simulink model "wlan_agc"  (Simulink 7.8)
settings: Solver=VariableStepDiscrete  SolverMode=SingleTasking  StartTime=0.0  StopTime=1e4  RelTol=1e-3
PostLoadFcn:
  | wlan_agc_init
InitFcn:
  | wlan_agc_init
StartFcn:
  | wlan_agc_init
values from neighbouring files (symbols this model uses):
  PHY_CONFIG_PKT_DET_CORR_THRESH = 90    [wlan_agc_init.m]
  PHY_CONFIG_PKT_DET_ENERGY_THRESH = 1    [wlan_agc_init.m]
  PHY_CONFIG_PKT_DET_MIN_DURR = 4    [wlan_agc_init.m]
undefined symbols (not defined in the file or in its folder): gcbh, xlBlockLoadCallback, xlGetNormalizedPeriod
libraries: xbsIndex_r4 x991, xbsEDKLib_r4 x1, simulink x1
(part 3 of 7)

== system wlan_agc/Gain Calc A ==
  I : Inport
  Q : Inport  Port=2
  IQ Valid : Inport  Port=3
  RSSI : Inport  Port=4
  BB gain : Subsystem
  Capture & Convert : Subsystem
  IQ Mag : Subsystem
  RF Gain : Subsystem
  RSSI Avg : Subsystem
  Register{1..4} (4 alike) : xbsIndex_r4/Register  init=0  rst=off  en=off  dbl_ovrd=off  block_type=register
  G_RF : Outport
  G_BB : Outport  Port=2
  wires:
  RF Gain/1(G_RF) -> Register1/1, Capture & Convert/1(G_RF)
  Register1/1 -> Register2/1
  RSSI/1 -> RSSI Avg/1(RSSI)
  RSSI Avg/1(avg) -> Capture & Convert/2(RSSI)
  Capture & Convert/1(Rx Pwr (dBm)) -> RF Gain/1(Rx Pwr), BB gain/2(P_IN_RSSI)
  Register3/1 -> Register4/1
  BB gain/1(G_BB) -> Register3/1
  RF Gain/2(G_RF_dB) -> BB gain/1(G_RF_dB)
  IQ Mag/1(IQ_dBv) -> BB gain/3(IQ_dBv)
  I/1 -> IQ Mag/1(I)
  Q/1 -> IQ Mag/2(Q)
  IQ Valid/1 -> IQ Mag/3(Valid)
  Register2/1 -> G_RF/1
  Register4/1 -> G_BB/1

== system wlan_agc/Gain Calc B ==
  I : Inport
  Q : Inport  Port=2
  IQ Valid : Inport  Port=3
  RSSI : Inport  Port=4
  BB gain : Subsystem
  Capture & Convert : Subsystem
  IQ Mag : Subsystem
  RF Gain : Subsystem
  RSSI Avg : Subsystem
  Register{1..4} (4 alike) : xbsIndex_r4/Register  init=0  rst=off  en=off  dbl_ovrd=off  block_type=register
  G_RF : Outport
  G_BB : Outport  Port=2
  wires:
  Register4/1 -> G_BB/1
  Register2/1 -> G_RF/1
  IQ Valid/1 -> IQ Mag/3(Valid)
  Q/1 -> IQ Mag/2(Q)
  I/1 -> IQ Mag/1(I)
  IQ Mag/1(IQ_dBv) -> BB gain/3(IQ_dBv)
  RF Gain/2(G_RF_dB) -> BB gain/1(G_RF_dB)
  BB gain/1(G_BB) -> Register3/1
  Register3/1 -> Register4/1
  Capture & Convert/1(Rx Pwr (dBm)) -> BB gain/2(P_IN_RSSI), RF Gain/1(Rx Pwr)
  RSSI Avg/1(avg) -> Capture & Convert/2(RSSI)
  RSSI/1 -> RSSI Avg/1(RSSI)
  Register1/1 -> Register2/1
  RF Gain/1(G_RF) -> Capture & Convert/1(G_RF), Register1/1

== system wlan_agc/Gain Calc C ==
  I : Inport
  Q : Inport  Port=2
  IQ Valid : Inport  Port=3
  RSSI : Inport  Port=4
  BB gain : Subsystem
  Capture & Convert : Subsystem
  IQ Mag : Subsystem
  RF Gain : Subsystem
  RSSI Avg : Subsystem
  Register{1..4} (4 alike) : xbsIndex_r4/Register  init=0  rst=off  en=off  dbl_ovrd=off  block_type=register
  G_RF : Outport
  G_BB : Outport  Port=2
  wires:
  RF Gain/1(G_RF) -> Register1/1, Capture & Convert/1(G_RF)
  Register1/1 -> Register2/1
  RSSI/1 -> RSSI Avg/1(RSSI)
  RSSI Avg/1(avg) -> Capture & Convert/2(RSSI)
  Capture & Convert/1(Rx Pwr (dBm)) -> RF Gain/1(Rx Pwr), BB gain/2(P_IN_RSSI)
  Register3/1 -> Register4/1
  BB gain/1(G_BB) -> Register3/1
  RF Gain/2(G_RF_dB) -> BB gain/1(G_RF_dB)
  IQ Mag/1(IQ_dBv) -> BB gain/3(IQ_dBv)
  I/1 -> IQ Mag/1(I)
  Q/1 -> IQ Mag/2(Q)
  IQ Valid/1 -> IQ Mag/3(Valid)
  Register2/1 -> G_RF/1
  Register4/1 -> G_BB/1

== system wlan_agc/Gain Calc D ==
  I : Inport
  Q : Inport  Port=2
  IQ Valid : Inport  Port=3
  RSSI : Inport  Port=4
  BB gain : Subsystem
  Capture & Convert : Subsystem
  IQ Mag : Subsystem
  RF Gain : Subsystem
  RSSI Avg : Subsystem
  Register{1..4} (4 alike) : xbsIndex_r4/Register  init=0  rst=off  en=off  dbl_ovrd=off  block_type=register
  G_RF : Outport
  G_BB : Outport  Port=2
  wires:
  Register4/1 -> G_BB/1
  Register2/1 -> G_RF/1
  IQ Valid/1 -> IQ Mag/3(Valid)
  Q/1 -> IQ Mag/2(Q)
  I/1 -> IQ Mag/1(I)
  IQ Mag/1(IQ_dBv) -> BB gain/3(IQ_dBv)
  RF Gain/2(G_RF_dB) -> BB gain/1(G_RF_dB)
  BB gain/1(G_BB) -> Register3/1
  Register3/1 -> Register4/1
  Capture & Convert/1(Rx Pwr (dBm)) -> BB gain/2(P_IN_RSSI), RF Gain/1(Rx Pwr)
  RSSI Avg/1(avg) -> Capture & Convert/2(RSSI)
  RSSI/1 -> RSSI Avg/1(RSSI)
  Register1/1 -> Register2/1
  RF Gain/1(G_RF) -> Capture & Convert/1(G_RF), Register1/1

== system wlan_agc/IQ Outputs ==
  IQ Valid : Inport
  A I : Inport  Port=2
  A Q : Inport  Port=3
  B I : Inport  Port=4
  B Q : Inport  Port=5
  C I : Inport  Port=6
  C Q : Inport  Port=7
  D I : Inport  Port=8
  D Q : Inport  Port=9
  IQ_Valid_Out : xbsIndex_r4/Gateway Out  inherit_from_input=off  hdl_port=on  timing_constraint=None  locs_specified=off  LOCs={}  UseAsDAC=off  DACChannel='1'  block_type=gatewayout
  RFA_RX_I_OUT : xbsIndex_r4/Gateway Out  inherit_from_input=off  hdl_port=on  timing_constraint=None  locs_specified=off  LOCs={}  UseAsDAC=off  DACChannel='1'  block_type=gatewayout
  RFA_RX_Q_OUT : xbsIndex_r4/Gateway Out  inherit_from_input=off  hdl_port=on  timing_constraint=None  locs_specified=off  LOCs={}  UseAsDAC=off  DACChannel='1'  block_type=gatewayout
  RFB_RX_I_OUT : xbsIndex_r4/Gateway Out  inherit_from_input=off  hdl_port=on  timing_constraint=None  locs_specified=off  LOCs={}  UseAsDAC=off  DACChannel='1'  block_type=gatewayout
  RFB_RX_Q_OUT : xbsIndex_r4/Gateway Out  inherit_from_input=off  hdl_port=on  timing_constraint=None  locs_specified=off  LOCs={}  UseAsDAC=off  DACChannel='1'  block_type=gatewayout
  RFC_RX_I_OUT : xbsIndex_r4/Gateway Out  inherit_from_input=off  hdl_port=on  timing_constraint=None  locs_specified=off  LOCs={}  UseAsDAC=off  DACChannel='1'  block_type=gatewayout
  RFC_RX_Q_OUT : xbsIndex_r4/Gateway Out  inherit_from_input=off  hdl_port=on  timing_constraint=None  locs_specified=off  LOCs={}  UseAsDAC=off  DACChannel='1'  block_type=gatewayout
  RFD_RX_I_OUT : xbsIndex_r4/Gateway Out  inherit_from_input=off  hdl_port=on  timing_constraint=None  locs_specified=off  LOCs={}  UseAsDAC=off  DACChannel='1'  block_type=gatewayout
  RFD_RX_Q_OUT : xbsIndex_r4/Gateway Out  inherit_from_input=off  hdl_port=on  timing_constraint=None  locs_specified=off  LOCs={}  UseAsDAC=off  DACChannel='1'  block_type=gatewayout
  wires:
  A I/1 -> RFA_RX_I_OUT/1
  A Q/1 -> RFA_RX_Q_OUT/1
  IQ Valid/1 -> IQ_Valid_Out/1
  B I/1 -> RFB_RX_I_OUT/1
  B Q/1 -> RFB_RX_Q_OUT/1
  C I/1 -> RFC_RX_I_OUT/1
  C Q/1 -> RFC_RX_Q_OUT/1
  D I/1 -> RFD_RX_I_OUT/1
  D Q/1 -> RFD_RX_Q_OUT/1

== system wlan_agc/RSSI Src ==
  Add : Sum
  Band-Limited White Noise : simulink/Sources/Band-Limited White Noise  Cov=200  Ts=1  seed=abs(ceil(1000*randn))
  Constant : Constant  Value=750
  Down Sample{,1..3} (4 alike) : xbsIndex_r4/Down Sample  sample_ratio=16  sample_phase="Last Value of Frame  (most efficient)"  en=off  latency=1  dbl_ovrd=off  block_type=dsamp
  RFA_RSSI : xbsIndex_r4/Gateway In  gui_display_data_type=Fixed-point  arith_type=Unsigned  n_bits=10  bin_pt=0  preci_type=Single  exp_width=8  frac_width=24  quantization="Round  (unbiased: +/- Inf)"  overflow=Saturate  period=1  dbl_ovrd=off  timing_constraint=None  locs_specified=off  LOCs={}  UseAsADC=off  ADCChannel='1'  inherit_from_input=off  hdl_port=on  block_type=gatewayin
  RFB_RSSI : xbsIndex_r4/Gateway In  gui_display_data_type=Fixed-point  arith_type=Unsigned  n_bits=10  bin_pt=0  preci_type=Single  exp_width=8  frac_width=24  quantization="Round  (unbiased: +/- Inf)"  overflow=Saturate  period=1  dbl_ovrd=off  timing_constraint=None  locs_specified=off  LOCs={}  UseAsADC=off  ADCChannel='1'  inherit_from_input=off  hdl_port=on  block_type=gatewayin
  RFC_RSSI : xbsIndex_r4/Gateway In  gui_display_data_type=Fixed-point  arith_type=Unsigned  n_bits=10  bin_pt=0  preci_type=Single  exp_width=8  frac_width=24  quantization="Round  (unbiased: +/- Inf)"  overflow=Saturate  period=1  dbl_ovrd=off  timing_constraint=None  locs_specified=off  LOCs={}  UseAsADC=off  ADCChannel='1'  inherit_from_input=off  hdl_port=on  block_type=gatewayin
  RFD_RSSI : xbsIndex_r4/Gateway In  gui_display_data_type=Fixed-point  arith_type=Unsigned  n_bits=10  bin_pt=0  preci_type=Single  exp_width=8  frac_width=24  quantization="Round  (unbiased: +/- Inf)"  overflow=Saturate  period=1  dbl_ovrd=off  timing_constraint=None  locs_specified=off  LOCs={}  UseAsADC=off  ADCChannel='1'  inherit_from_input=off  hdl_port=on  block_type=gatewayin
  Register{,1..3} (4 alike) : xbsIndex_r4/Register  init=0  rst=off  en=off  dbl_ovrd=off  block_type=register
  " RFA_RSSI" : Outport
  " RFB_RSSI" : Outport  Port=2
  " RFC_RSSI" : Outport  Port=3
  " RFD_RSSI" : Outport  Port=4
  wires:
  RFA_RSSI/1 -> Register/1
  Register/1 -> Down Sample/1
  Down Sample/1 -> " RFA_RSSI"/1
  Add/1 -> RFA_RSSI/1, RFB_RSSI/1, RFC_RSSI/1, RFD_RSSI/1
  Constant/1 -> Add/1
  Band-Limited White Noise/1 -> Add/2
  RFB_RSSI/1 -> Register1/1
  Register1/1 -> Down Sample1/1
  Down Sample1/1 -> " RFB_RSSI"/1
  RFC_RSSI/1 -> Register2/1
  RFD_RSSI/1 -> Register3/1
  Register2/1 -> Down Sample2/1
  Register3/1 -> Down Sample3/1
  Down Sample3/1 -> " RFD_RSSI"/1
  Down Sample2/1 -> " RFC_RSSI"/1

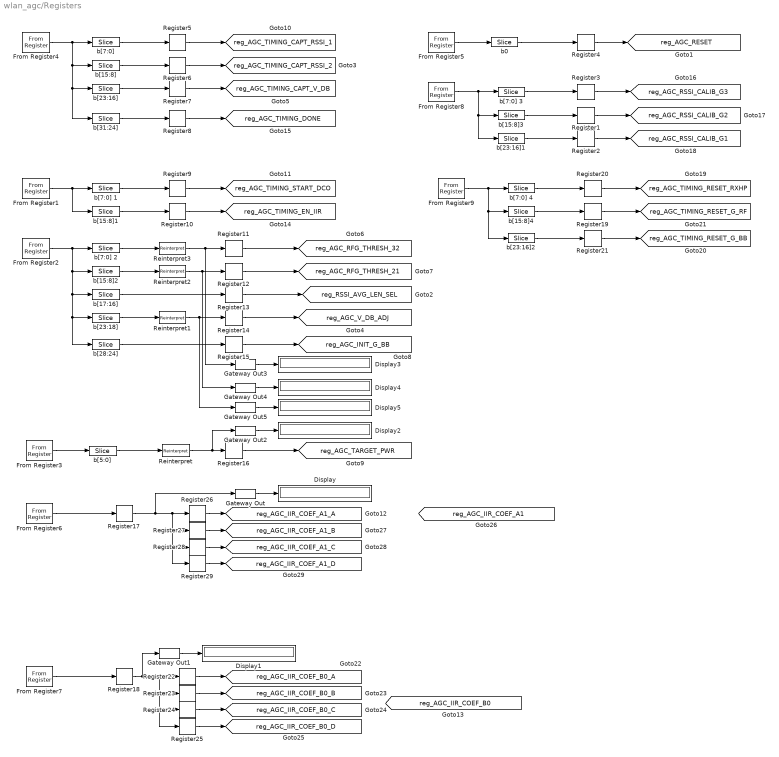
== system wlan_agc/Registers ==
  Display{,1..5} (6 alike) : Display
  From Register1 : xbsIndex_r4/From Register  shared_memory_name='TIMING_DCO'  init=REG_AGC_Timing_DCO  period=1  ownership=Locally owned and initialized  gui_display_data_type=Fixed-point  arith_type=Unsigned  n_bits=32  bin_pt=0  preci_type=Single  dbl_ovrd=off  block_type=fromreg
      settings: AttributesFormatString=<< %<shared_memory_name> >>  infoedit="Register block that reads data to a shared memory register.  Delay of one sample period."
  From Register2 : xbsIndex_r4/From Register  shared_memory_name='CONFIG'  init=REG_AGC_Config  period=1  ownership=Locally owned and initialized  gui_display_data_type=Fixed-point  arith_type=Unsigned  n_bits=32  bin_pt=0  preci_type=Single  dbl_ovrd=off  block_type=fromreg
      settings: AttributesFormatString=<< %<shared_memory_name> >>  infoedit="Register block that reads data to a shared memory register.  Delay of one sample period."
  From Register3 : xbsIndex_r4/From Register  shared_memory_name='TARGET'  init=REG_AGC_Target  period=1  ownership=Locally owned and initialized  gui_display_data_type=Fixed-point  arith_type=Unsigned  n_bits=32  bin_pt=0  preci_type=Single  dbl_ovrd=off  block_type=fromreg
      settings: AttributesFormatString=<< %<shared_memory_name> >>  infoedit="Register block that reads data to a shared memory register.  Delay of one sample period."
  From Register4 : xbsIndex_r4/From Register  shared_memory_name='TIMING_AGC'  init=REG_AGC_Timing_AGC  period=1  ownership=Locally owned and initialized  gui_display_data_type=Fixed-point  arith_type=Unsigned  n_bits=32  bin_pt=0  preci_type=Single  dbl_ovrd=off  block_type=fromreg
      settings: AttributesFormatString=<< %<shared_memory_name> >>  infoedit="Register block that reads data to a shared memory register.  Delay of one sample period."
  From Register5 : xbsIndex_r4/From Register  shared_memory_name='RESET'  init=0  period=1  ownership=Locally owned and initialized  gui_display_data_type=Fixed-point  arith_type=Unsigned  n_bits=32  bin_pt=0  preci_type=Single  dbl_ovrd=off  block_type=fromreg
      settings: AttributesFormatString=<< %<shared_memory_name> >>  infoedit="Register block that reads data to a shared memory register.  Delay of one sample period."
  From Register6 : xbsIndex_r4/From Register  shared_memory_name='IIR_COEF_A1'  init=REG_AGC_IIR_Coef_A1  period=1  ownership=Locally owned and initialized  gui_display_data_type=Fixed-point  arith_type="Signed  (2's comp)"  n_bits=18  bin_pt=17  preci_type=Single  dbl_ovrd=off  block_type=fromreg
      settings: AttributesFormatString=<< %<shared_memory_name> >>  infoedit="Register block that reads data to a shared memory register.  Delay of one sample period."
  From Register7 : xbsIndex_r4/From Register  shared_memory_name='IIR_COEF_B0'  init=REG_AGC_IIR_Coef_B0  period=1  ownership=Locally owned and initialized  gui_display_data_type=Fixed-point  arith_type=Unsigned  n_bits=18  bin_pt=17  preci_type=Single  dbl_ovrd=off  block_type=fromreg
      settings: AttributesFormatString=<< %<shared_memory_name> >>  infoedit="Register block that reads data to a shared memory register.  Delay of one sample period."
  From Register8 : xbsIndex_r4/From Register  shared_memory_name='RSSI_PWR_CALIB'  init=REG_AGC_RSSI_RX_PWR_CALIB  period=1  ownership=Locally owned and initialized  gui_display_data_type=Fixed-point  arith_type=Unsigned  n_bits=32  bin_pt=0  preci_type=Single  dbl_ovrd=off  block_type=fromreg
      settings: AttributesFormatString=<< %<shared_memory_name> >>  infoedit="Register block that reads data to a shared memory register.  Delay of one sample period."
  From Register9 : xbsIndex_r4/From Register  shared_memory_name='TIMING_RESET'  init=REG_AGC_Timing_Reset  period=1  ownership=Locally owned and initialized  gui_display_data_type=Fixed-point  arith_type=Unsigned  n_bits=32  bin_pt=0  preci_type=Single  dbl_ovrd=off  block_type=fromreg
      settings: AttributesFormatString=<< %<shared_memory_name> >>  infoedit="Register block that reads data to a shared memory register.  Delay of one sample period."
  Gateway Out{,1..5} (6 alike) : xbsIndex_r4/Gateway Out  inherit_from_input=off  hdl_port=off  timing_constraint=None  locs_specified=off  LOCs={}  UseAsDAC=off  DACChannel='1'  block_type=gatewayout
  Register{1..29} (29 alike) : xbsIndex_r4/Register  init=0  rst=off  en=off  dbl_ovrd=off  block_type=register
  Reinterpret{,1..3} (4 alike) : xbsIndex_r4/Reinterpret  force_arith_type=on  arith_type="Signed  (2's comp)"  force_bin_pt=off  bin_pt=0  block_type=reinterpret
  b0 : xbsIndex_r4/Slice  nbits=1  boolean_output=on  mode=Lower Bit Location + Width  bit1=0  base1=MSB of Input  bit0=0  base0=LSB of Input  dbl_ovrd=off  block_type=slice
      settings: block_version=VER_STRING_GOES_HERE
  b[15:8]{,1..4} (5 alike) : xbsIndex_r4/Slice  nbits=8  boolean_output=off  mode=Lower Bit Location + Width  bit1=0  base1=MSB of Input  bit0=8  base0=LSB of Input  dbl_ovrd=off  block_type=slice
      settings: block_version=VER_STRING_GOES_HERE
  b[17:16] : xbsIndex_r4/Slice  nbits=2  boolean_output=off  mode=Lower Bit Location + Width  bit1=0  base1=MSB of Input  bit0=16  base0=LSB of Input  dbl_ovrd=off  block_type=slice
      settings: block_version=VER_STRING_GOES_HERE
  b[23:16] : xbsIndex_r4/Slice  nbits=8  boolean_output=off  mode=Lower Bit Location + Width  bit1=0  base1=MSB of Input  bit0=16  base0=LSB of Input  dbl_ovrd=off  block_type=slice
      settings: block_version=VER_STRING_GOES_HERE
  b[23:16]1 : xbsIndex_r4/Slice  nbits=8  boolean_output=off  mode=Lower Bit Location + Width  bit1=0  base1=MSB of Input  bit0=16  base0=LSB of Input  dbl_ovrd=off  block_type=slice
      settings: block_version=VER_STRING_GOES_HERE
  b[23:16]2 : xbsIndex_r4/Slice  nbits=8  boolean_output=off  mode=Lower Bit Location + Width  bit1=0  base1=MSB of Input  bit0=16  base0=LSB of Input  dbl_ovrd=off  block_type=slice
      settings: block_version=VER_STRING_GOES_HERE
  b[23:18] : xbsIndex_r4/Slice  nbits=6  boolean_output=off  mode=Lower Bit Location + Width  bit1=0  base1=MSB of Input  bit0=18  base0=LSB of Input  dbl_ovrd=off  block_type=slice
      settings: block_version=VER_STRING_GOES_HERE
  b[28:24] : xbsIndex_r4/Slice  nbits=5  boolean_output=off  mode=Lower Bit Location + Width  bit1=0  base1=MSB of Input  bit0=24  base0=LSB of Input  dbl_ovrd=off  block_type=slice
      settings: block_version=VER_STRING_GOES_HERE
  b[31:24] : xbsIndex_r4/Slice  nbits=8  boolean_output=off  mode=Lower Bit Location + Width  bit1=0  base1=MSB of Input  bit0=24  base0=LSB of Input  dbl_ovrd=off  block_type=slice
      settings: block_version=VER_STRING_GOES_HERE
  b[5:0] : xbsIndex_r4/Slice  nbits=6  boolean_output=off  mode=Lower Bit Location + Width  bit1=0  base1=MSB of Input  bit0=0  base0=LSB of Input  dbl_ovrd=off  block_type=slice
      settings: block_version=VER_STRING_GOES_HERE
  b[7:0] {,1..4} (5 alike) : xbsIndex_r4/Slice  nbits=8  boolean_output=off  mode=Lower Bit Location + Width  bit1=0  base1=MSB of Input  bit0=0  base0=LSB of Input  dbl_ovrd=off  block_type=slice
      settings: block_version=VER_STRING_GOES_HERE
  tag scope: reg_AGC_IIR_COEF_A1=global, reg_AGC_IIR_COEF_A1_A=global, reg_AGC_IIR_COEF_A1_B=global, reg_AGC_IIR_COEF_A1_C=global, reg_AGC_IIR_COEF_A1_D=global, reg_AGC_IIR_COEF_B0=global, reg_AGC_IIR_COEF_B0_A=global, reg_AGC_IIR_COEF_B0_B=global, reg_AGC_IIR_COEF_B0_C=global, reg_AGC_IIR_COEF_B0_D=global, reg_AGC_INIT_G_BB=global, reg_AGC_RESET=global, reg_AGC_RFG_THRESH_21=global, reg_AGC_RFG_THRESH_32=global, reg_AGC_RSSI_CALIB_G1=global, reg_AGC_RSSI_CALIB_G2=global, reg_AGC_RSSI_CALIB_G3=global, reg_AGC_TARGET_PWR=global, reg_AGC_TIMING_CAPT_RSSI_1=global, reg_AGC_TIMING_CAPT_RSSI_2=global, reg_AGC_TIMING_CAPT_V_DB=global, reg_AGC_TIMING_DONE=global, reg_AGC_TIMING_EN_IIR=global, reg_AGC_TIMING_RESET_G_BB=global, reg_AGC_TIMING_RESET_G_RF=global, reg_AGC_TIMING_RESET_RXHP=global, reg_AGC_TIMING_START_DCO=global, reg_AGC_V_DB_ADJ=global, reg_RSSI_AVG_LEN_SEL=global
  wires:
  From Register4/1 -> "b[7:0] "/1, b[15:8]/1, b[23:16]/1, b[31:24]/1
  "b[7:0] "/1 -> Register5/1
  b[15:8]/1 -> Register6/1
  b[23:16]/1 -> Register7/1
  From Register1/1 -> b[7:0] 1/1, b[15:8]1/1
  b[7:0] 1/1 -> Register9/1
  b[15:8]1/1 -> Register10/1
  From Register2/1 -> b[15:8]2/1, b[17:16]/1, b[23:18]/1, b[28:24]/1, b[7:0] 2/1
  b[7:0] 2/1 -> Reinterpret3/1
  b[15:8]2/1 -> Reinterpret2/1
  b[17:16]/1 -> Register13/1
  b[23:18]/1 -> Reinterpret1/1
  b[28:24]/1 -> Register15/1
  From Register3/1 -> b[5:0]/1
  b[5:0]/1 -> Reinterpret/1
  Reinterpret/1 -> Gateway Out2/1, Register16/1
  Reinterpret1/1 -> Gateway Out5/1, Register14/1
  Reinterpret2/1 -> Gateway Out4/1, Register12/1
  Reinterpret3/1 -> Gateway Out3/1, Register11/1
  From Register5/1 -> b0/1
  b0/1 -> Register4/1
  From Register6/1 -> Register17/1
  From Register7/1 -> Register18/1
  Gateway Out/1 -> Display/1
  Gateway Out1/1 -> Display1/1
  Gateway Out2/1 -> Display2/1
  Gateway Out3/1 -> Display3/1
  Gateway Out4/1 -> Display4/1
  Gateway Out5/1 -> Display5/1
  b[31:24]/1 -> Register8/1
  From Register8/1 -> b[15:8]3/1, b[23:16]1/1, b[7:0] 3/1
  b[7:0] 3/1 -> Register3/1
  b[15:8]3/1 -> Register1/1
  b[23:16]1/1 -> Register2/1
  Register3/1 -> [reg_AGC_RSSI_CALIB_G3]
  Register1/1 -> [reg_AGC_RSSI_CALIB_G2]
  Register2/1 -> [reg_AGC_RSSI_CALIB_G1]
  Register4/1 -> [reg_AGC_RESET]
  Register5/1 -> [reg_AGC_TIMING_CAPT_RSSI_1]
  Register6/1 -> [reg_AGC_TIMING_CAPT_RSSI_2]
  Register7/1 -> [reg_AGC_TIMING_CAPT_V_DB]
  Register8/1 -> [reg_AGC_TIMING_DONE]
  Register9/1 -> [reg_AGC_TIMING_START_DCO]
  Register10/1 -> [reg_AGC_TIMING_EN_IIR]
  Register11/1 -> [reg_AGC_RFG_THRESH_32]
  Register12/1 -> [reg_AGC_RFG_THRESH_21]
  Register13/1 -> [reg_RSSI_AVG_LEN_SEL]
  Register14/1 -> [reg_AGC_V_DB_ADJ]
  Register15/1 -> [reg_AGC_INIT_G_BB]
  Register16/1 -> [reg_AGC_TARGET_PWR]
  Register17/1 -> Gateway Out/1, Register28/1, Register29/1, Register27/1, Register26/1
  Register18/1 -> Gateway Out1/1, Register24/1, Register25/1, Register23/1, Register22/1
  From Register9/1 -> b[7:0] 4/1, b[15:8]4/1, b[23:16]2/1
  b[7:0] 4/1 -> Register20/1
  b[15:8]4/1 -> Register19/1
  Register20/1 -> [reg_AGC_TIMING_RESET_RXHP]
  Register19/1 -> [reg_AGC_TIMING_RESET_G_RF]
  b[23:16]2/1 -> Register21/1
  Register21/1 -> [reg_AGC_TIMING_RESET_G_BB]
  Register22/1 -> [reg_AGC_IIR_COEF_B0_A]
  Register23/1 -> [reg_AGC_IIR_COEF_B0_B]
  Register24/1 -> [reg_AGC_IIR_COEF_B0_C]
  Register25/1 -> [reg_AGC_IIR_COEF_B0_D]
  Register26/1 -> [reg_AGC_IIR_COEF_A1_A]
  Register27/1 -> [reg_AGC_IIR_COEF_A1_B]
  Register28/1 -> [reg_AGC_IIR_COEF_A1_C]
  Register29/1 -> [reg_AGC_IIR_COEF_A1_D]

== system wlan_agc/S-R Latch ==
  S : Inport
  R : Inport  Port=2
  Constant1 : xbsIndex_r4/Constant  const=1  gui_display_data_type=Boolean  arith_type=Boolean  n_bits=1  bin_pt=0  preci_type=Single  exp_width=8  frac_width=24  explicit_period=off  period=1  equ=P=C  opselect=C  inp2=PCIN>>17  opr=+  inp1=P  carry=CIN  dbl_ovrd=off  block_type=constant
      settings: block_version=VER_STRING_GOES_HERE
  Convert1 : xbsIndex_r4/Convert  gui_display_data_type=Boolean  arith_type=Boolean  n_bits=1  bin_pt=0  float_type=Single  exp_bits=8  fraction_bits=24  quantization=Truncate  overflow=Wrap  en=off  latency=0  dbl_ovrd=off  pipeline=off  block_type=convert
  Convert2 : xbsIndex_r4/Convert  gui_display_data_type=Boolean  arith_type=Boolean  n_bits=1  bin_pt=0  float_type=Single  exp_bits=8  fraction_bits=24  quantization=Truncate  overflow=Wrap  en=off  latency=0  dbl_ovrd=off  pipeline=off  block_type=convert
  Register2 : xbsIndex_r4/Register  init=0  rst=on  en=on  dbl_ovrd=off  block_type=register
      settings: xl_area=[1 1 0 0 0 0 0]  block_version=VER_STRING_GOES_HERE
  Q : Outport
  wires:
  Convert2/1 -> Register2/3
  Convert1/1 -> Register2/2
  Constant1/1 -> Register2/1
  R/1 -> Convert1/1
  Register2/1 -> Q/1
  S/1 -> Convert2/1

== system wlan_agc/Auto-Corr Pkt Det/Auto Corr ==
  Valid : Inport
  I : Inport  Port=2
  Q : Inport  Port=3
  Avg Mag : Subsystem
  Conj Mult : Subsystem
  Delay : xbsIndex_r4/Delay  rst=off  infoeditControl=Selection of Reset will increase slice count due to use of real FFs and instead of SRLs  en=on  latency=16  dbl_ovrd=off  reg_retiming=off  block_type=delay
      settings: xl_area=[7 14 0 14 0 0 0]  block_version=VER_STRING_GOES_HERE
  Delay1 : xbsIndex_r4/Delay  rst=off  infoeditControl=Selection of Reset will increase slice count due to use of real FFs and instead of SRLs  en=on  latency=16  dbl_ovrd=off  reg_retiming=off  block_type=delay
      settings: xl_area=[7 14 0 14 0 0 0]  block_version=VER_STRING_GOES_HERE
  Corr : Outport
  wires:
  I/1 -> Delay/1, Conj Mult/2(A I)
  Q/1 -> Delay1/1, Conj Mult/3(A Q)
  Delay/1 -> Conj Mult/4(B I)
  Delay1/1 -> Conj Mult/5(B Q)
  Valid/1 -> Conj Mult/1(Valid), Delay1/2, Delay/2
  Conj Mult/2(" I") -> Avg Mag/2(I)
  Conj Mult/3(" Q") -> Avg Mag/3(Q)
  Conj Mult/1(" Valid") -> Avg Mag/1(Valid)
  Avg Mag/1(M) -> Corr/1

== system wlan_agc/Auto-Corr Pkt Det/Decision ==
  PktDet Reset : Inport
  Corr : Inport  Port=2
  Mag : Inport  Port=3
  Display{,1..3} (4 alike) : Display
  Logical : xbsIndex_r4/Logical  logical_function=AND  inputs=2  en=off  latency=0  precision=Full  arith_type=Unsigned  n_bits=8  bin_pt=2  align_bp=on  dbl_ovrd=off  block_type=logical
      settings: xl_area=[1 0 0 1 0 0 0]  block_version=VER_STRING_GOES_HERE
  Min Dur : Subsystem
  Mult1 : xbsIndex_r4/Mult  precision=User Defined  arith_type=Unsigned  n_bits=30  bin_pt=20  quantization=Truncate  overflow=Flag as error  en=off  latency=1  dbl_ovrd=off  use_behavioral_HDL=off  opt=Speed  use_embedded=on  optimum_pipeline=off  pipeline=on  use_rpm=off  placement_style=Rectangular shape  block_type=mult
      settings: xl_area=[63 105 0 106 0 4 0]  block_version=VER_STRING_GOES_HERE
  Reinterpret : xbsIndex_r4/Reinterpret  force_arith_type=on  arith_type=Unsigned  force_bin_pt=on  bin_pt=0  block_type=reinterpret
  Reinterpret1 : xbsIndex_r4/Reinterpret  force_arith_type=on  arith_type=Unsigned  force_bin_pt=on  bin_pt=0  block_type=reinterpret
  Relational : xbsIndex_r4/Relational  mode=a>b  en=off  latency=1  dbl_ovrd=off  block_type=relational
      settings: xl_area=[11 1 0 22 0 0 0]  block_version=VER_STRING_GOES_HERE
  Relational1 : xbsIndex_r4/Relational  mode=a>b  en=off  latency=1  dbl_ovrd=off  block_type=relational
      settings: xl_area=[11 1 0 22 0 0 0]  block_version=VER_STRING_GOES_HERE
  done{14..15,17..18} (4 alike) : xbsIndex_r4/Gateway Out  inherit_from_input=off  hdl_port=off  timing_constraint=None  locs_specified=off  LOCs={}  UseAsDAC=off  DACChannel='1'  block_type=gatewayout
      settings: infoedit="Gateway out block.  Converts Xilinx fixed point inputs into ouputs of type Simulink integer, double, or fixed point.<P><P>Hardware notes:  In hardware these blocks become top level output ports or are discarded, depending on how they are configured."  xl_area=[0 0 0 0 1 0 0]  block_version=VER_STRING_GOES_HERE
  PktDet : Outport
  wires:
  done18/1 -> Display3/1
  Reinterpret1/1 -> done18/1
  done17/1 -> Display2/1
  Reinterpret/1 -> done17/1
  done15/1 -> Display1/1
  done14/1 -> Display/1
  [regRx_PktDet_CorrThresh] -> Reinterpret/1, done14/1
  [regRx_PktDet_EnergyThresh] -> Reinterpret1/1, done15/1
  Corr/1 -> Relational/1
  Mag/1 -> Mult1/2, Relational1/1
  [regRx_PktDet_CorrThresh] -> Mult1/1
  Mult1/1 -> Relational/2
  [regRx_PktDet_EnergyThresh] -> Relational1/2
  Logical/1 -> Min Dur/1(Det)
  PktDet Reset/1 -> Min Dur/2(Reset)
  Min Dur/1(Pkt Det) -> PktDet/1
  Relational/1 -> Logical/1
  Relational1/1 -> Logical/2

== system wlan_agc/Auto-Corr Pkt Det/Mag ==
  Valid : Inport
  I : Inport  Port=2
  Q : Inport  Port=3
  AddSub : xbsIndex_r4/AddSub  mode=Addition  use_carryin=off  use_carryout=off  en=off  latency=0  precision=User Defined  arith_type="Signed  (2's comp)"  n_bits=20  bin_pt=18  quantization=Truncate  overflow=Flag as error  dbl_ovrd=off  use_behavioral_HDL=off  hw_selection=Fabric  pipelined=off  block_type=addsub
  Delay : xbsIndex_r4/Delay  rst=off  infoeditControl=Selection of Reset will increase slice count due to use of real FFs and instead of SRLs  en=off  latency=1  dbl_ovrd=off  reg_retiming=off  block_type=delay
  Mult : xbsIndex_r4/Mult  precision=User Defined  arith_type="Signed  (2's comp)"  n_bits=20  bin_pt=19  quantization=Truncate  overflow=Saturate  en=off  latency=1  dbl_ovrd=off  use_behavioral_HDL=off  opt=Speed  use_embedded=on  optimum_pipeline=off  pipeline=on  use_rpm=on  placement_style=Triangular  block_type=mult
  Mult1 : xbsIndex_r4/Mult  precision=User Defined  arith_type="Signed  (2's comp)"  n_bits=20  bin_pt=19  quantization=Truncate  overflow=Saturate  en=off  latency=1  dbl_ovrd=off  use_behavioral_HDL=off  opt=Speed  use_embedded=on  optimum_pipeline=off  pipeline=on  use_rpm=on  placement_style=Triangular  block_type=mult
  Mult2 : xbsIndex_r4/Mult  precision=User Defined  arith_type="Signed  (2's comp)"  n_bits=25  bin_pt=18  quantization=Truncate  overflow=Saturate  en=on  latency=1  dbl_ovrd=off  use_behavioral_HDL=off  opt=Speed  use_embedded=on  optimum_pipeline=off  pipeline=on  use_rpm=on  placement_style=Triangular  block_type=mult
  Running Sum : Subsystem
  Mag Sq : Outport
  Mag : Outport  Port=2
  wires:
  Delay/1 -> Running Sum/1(En)
  I/1 -> Mult/1, Mult/2
  Valid/1 -> Delay/1
  Running Sum/1(Sum) -> Mult2/1, Mult2/2, Mag/1
  Q/1 -> Mult1/1, Mult1/2
  Mult/1 -> AddSub/1
  Mult1/1 -> AddSub/2
  AddSub/1 -> Running Sum/2(D)
  Mult2/1 -> Mag Sq/1
  Running Sum/2(Valid) -> Mult2/3

== system wlan_agc/Ctrl/Negedge ==
  D : Inport
  Delay : xbsIndex_r4/Delay  rst=off  infoeditControl=Selection of Reset will increase slice count due to use of real FFs and instead of SRLs  en=off  latency=1  dbl_ovrd=off  reg_retiming=off  block_type=delay
      settings: infoedit=Hardware notes: A delay line is a chain, each link of which is an SRL16 followed by a flip-flop. If register retiming is enabled, the delay line is a chain of flip-flops.  xl_area=[1 1 0 0 0 0 0]  block_version=VER_STRING_GOES_HERE
  Inverter : xbsIndex_r4/Inverter  en=off  latency=0  dbl_ovrd=off  block_type=inv
      settings: xl_area=[0 0 0 0 0 0 0]  block_version=VER_STRING_GOES_HERE
  Logical1 : xbsIndex_r4/Logical  logical_function=AND  inputs=2  en=off  latency=0  precision=Full  arith_type=Unsigned  n_bits=8  bin_pt=2  align_bp=on  dbl_ovrd=off  block_type=logical
      settings: xl_area=[1 0 0 1 0 0 0]  block_version=VER_STRING_GOES_HERE
  Q : Outport
  wires:
  Delay/1 -> Logical1/1
  Logical1/1 -> Q/1
  D/1 -> Delay/1, Inverter/1
  Inverter/1 -> Logical1/2

== system wlan_agc/Ctrl/Posedge1 ==
  note: Rising Edge Detection
  D : Inport
  Delay : xbsIndex_r4/Delay  rst=off  infoeditControl=Selection of Reset will increase slice count due to use of real FFs and instead of SRLs  en=off  latency=1  dbl_ovrd=off  reg_retiming=off  block_type=delay
      settings: infoedit=Hardware notes: A delay line is a chain, each link of which is an SRL16 followed by a flip-flop. If register retiming is enabled, the delay line is a chain of flip-flops.  xl_area=[1 1 0 0 0 0 0]  block_version=VER_STRING_GOES_HERE
  Inverter : xbsIndex_r4/Inverter  en=off  latency=0  dbl_ovrd=off  block_type=inv
      settings: xl_area=[0 0 0 0 0 0 0]  block_version=VER_STRING_GOES_HERE
  Logical1 : xbsIndex_r4/Logical  logical_function=AND  inputs=2  en=off  latency=0  precision=Full  arith_type=Unsigned  n_bits=8  bin_pt=2  align_bp=on  dbl_ovrd=off  block_type=logical
      settings: xl_area=[1 0 0 1 0 0 0]  block_version=VER_STRING_GOES_HERE
  Q : Outport
  wires:
  Delay/1 -> Inverter/1
  Inverter/1 -> Logical1/1
  Logical1/1 -> Q/1
  D/1 -> Delay/1, Logical1/2

== system wlan_agc/Ctrl/Posedge10 ==
  note: Rising Edge Detection
  D : Inport
  Delay : xbsIndex_r4/Delay  rst=off  infoeditControl=Selection of Reset will increase slice count due to use of real FFs and instead of SRLs  en=off  latency=1  dbl_ovrd=off  reg_retiming=off  block_type=delay
      settings: infoedit=Hardware notes: A delay line is a chain, each link of which is an SRL16 followed by a flip-flop. If register retiming is enabled, the delay line is a chain of flip-flops.  xl_area=[1 1 0 0 0 0 0]  block_version=VER_STRING_GOES_HERE
  Inverter : xbsIndex_r4/Inverter  en=off  latency=0  dbl_ovrd=off  block_type=inv
      settings: xl_area=[0 0 0 0 0 0 0]  block_version=VER_STRING_GOES_HERE
  Logical1 : xbsIndex_r4/Logical  logical_function=AND  inputs=2  en=off  latency=0  precision=Full  arith_type=Unsigned  n_bits=8  bin_pt=2  align_bp=on  dbl_ovrd=off  block_type=logical
      settings: xl_area=[1 0 0 1 0 0 0]  block_version=VER_STRING_GOES_HERE
  Q : Outport
  wires:
  D/1 -> Logical1/2, Delay/1
  Logical1/1 -> Q/1
  Inverter/1 -> Logical1/1
  Delay/1 -> Inverter/1

== system wlan_agc/Ctrl/Posedge2 ==
  note: Rising Edge Detection
  D : Inport
  Delay : xbsIndex_r4/Delay  rst=off  infoeditControl=Selection of Reset will increase slice count due to use of real FFs and instead of SRLs  en=off  latency=1  dbl_ovrd=off  reg_retiming=off  block_type=delay
      settings: infoedit=Hardware notes: A delay line is a chain, each link of which is an SRL16 followed by a flip-flop. If register retiming is enabled, the delay line is a chain of flip-flops.  xl_area=[1 1 0 0 0 0 0]  block_version=VER_STRING_GOES_HERE
  Inverter : xbsIndex_r4/Inverter  en=off  latency=0  dbl_ovrd=off  block_type=inv
      settings: xl_area=[0 0 0 0 0 0 0]  block_version=VER_STRING_GOES_HERE
  Logical1 : xbsIndex_r4/Logical  logical_function=AND  inputs=2  en=off  latency=0  precision=Full  arith_type=Unsigned  n_bits=8  bin_pt=2  align_bp=on  dbl_ovrd=off  block_type=logical
      settings: xl_area=[1 0 0 1 0 0 0]  block_version=VER_STRING_GOES_HERE
  Q : Outport
  wires:
  D/1 -> Logical1/2, Delay/1
  Logical1/1 -> Q/1
  Inverter/1 -> Logical1/1
  Delay/1 -> Inverter/1

== system wlan_agc/Ctrl/Posedge3 ==
  note: Rising Edge Detection
  D : Inport
  Delay : xbsIndex_r4/Delay  rst=off  infoeditControl=Selection of Reset will increase slice count due to use of real FFs and instead of SRLs  en=off  latency=1  dbl_ovrd=off  reg_retiming=off  block_type=delay
      settings: infoedit=Hardware notes: A delay line is a chain, each link of which is an SRL16 followed by a flip-flop. If register retiming is enabled, the delay line is a chain of flip-flops.  xl_area=[1 1 0 0 0 0 0]  block_version=VER_STRING_GOES_HERE
  Inverter : xbsIndex_r4/Inverter  en=off  latency=0  dbl_ovrd=off  block_type=inv
      settings: xl_area=[0 0 0 0 0 0 0]  block_version=VER_STRING_GOES_HERE
  Logical1 : xbsIndex_r4/Logical  logical_function=AND  inputs=2  en=off  latency=0  precision=Full  arith_type=Unsigned  n_bits=8  bin_pt=2  align_bp=on  dbl_ovrd=off  block_type=logical
      settings: xl_area=[1 0 0 1 0 0 0]  block_version=VER_STRING_GOES_HERE
  Q : Outport
  wires:
  D/1 -> Logical1/2, Delay/1
  Logical1/1 -> Q/1
  Inverter/1 -> Logical1/1
  Delay/1 -> Inverter/1

== system wlan_agc/Ctrl/Posedge4 ==
  note: Rising Edge Detection
  D : Inport
  Delay : xbsIndex_r4/Delay  rst=off  infoeditControl=Selection of Reset will increase slice count due to use of real FFs and instead of SRLs  en=off  latency=1  dbl_ovrd=off  reg_retiming=off  block_type=delay
      settings: infoedit=Hardware notes: A delay line is a chain, each link of which is an SRL16 followed by a flip-flop. If register retiming is enabled, the delay line is a chain of flip-flops.  xl_area=[1 1 0 0 0 0 0]  block_version=VER_STRING_GOES_HERE
  Inverter : xbsIndex_r4/Inverter  en=off  latency=0  dbl_ovrd=off  block_type=inv
      settings: xl_area=[0 0 0 0 0 0 0]  block_version=VER_STRING_GOES_HERE
  Logical1 : xbsIndex_r4/Logical  logical_function=AND  inputs=2  en=off  latency=0  precision=Full  arith_type=Unsigned  n_bits=8  bin_pt=2  align_bp=on  dbl_ovrd=off  block_type=logical
      settings: xl_area=[1 0 0 1 0 0 0]  block_version=VER_STRING_GOES_HERE
  Q : Outport
  wires:
  D/1 -> Logical1/2, Delay/1
  Logical1/1 -> Q/1
  Inverter/1 -> Logical1/1
  Delay/1 -> Inverter/1

== system wlan_agc/Ctrl/Posedge5 ==
  note: Rising Edge Detection
  D : Inport
  Delay : xbsIndex_r4/Delay  rst=off  infoeditControl=Selection of Reset will increase slice count due to use of real FFs and instead of SRLs  en=off  latency=1  dbl_ovrd=off  reg_retiming=off  block_type=delay
      settings: infoedit=Hardware notes: A delay line is a chain, each link of which is an SRL16 followed by a flip-flop. If register retiming is enabled, the delay line is a chain of flip-flops.  xl_area=[1 1 0 0 0 0 0]  block_version=VER_STRING_GOES_HERE
  Inverter : xbsIndex_r4/Inverter  en=off  latency=0  dbl_ovrd=off  block_type=inv
      settings: xl_area=[0 0 0 0 0 0 0]  block_version=VER_STRING_GOES_HERE
  Logical1 : xbsIndex_r4/Logical  logical_function=AND  inputs=2  en=off  latency=0  precision=Full  arith_type=Unsigned  n_bits=8  bin_pt=2  align_bp=on  dbl_ovrd=off  block_type=logical
      settings: xl_area=[1 0 0 1 0 0 0]  block_version=VER_STRING_GOES_HERE
  Q : Outport
  wires:
  D/1 -> Logical1/2, Delay/1
  Logical1/1 -> Q/1
  Inverter/1 -> Logical1/1
  Delay/1 -> Inverter/1

== system wlan_agc/Ctrl/Posedge6 ==
  note: Rising Edge Detection
  D : Inport
  Delay : xbsIndex_r4/Delay  rst=off  infoeditControl=Selection of Reset will increase slice count due to use of real FFs and instead of SRLs  en=off  latency=1  dbl_ovrd=off  reg_retiming=off  block_type=delay
      settings: infoedit=Hardware notes: A delay line is a chain, each link of which is an SRL16 followed by a flip-flop. If register retiming is enabled, the delay line is a chain of flip-flops.  xl_area=[1 1 0 0 0 0 0]  block_version=VER_STRING_GOES_HERE
  Inverter : xbsIndex_r4/Inverter  en=off  latency=0  dbl_ovrd=off  block_type=inv
      settings: xl_area=[0 0 0 0 0 0 0]  block_version=VER_STRING_GOES_HERE
  Logical1 : xbsIndex_r4/Logical  logical_function=AND  inputs=2  en=off  latency=0  precision=Full  arith_type=Unsigned  n_bits=8  bin_pt=2  align_bp=on  dbl_ovrd=off  block_type=logical
      settings: xl_area=[1 0 0 1 0 0 0]  block_version=VER_STRING_GOES_HERE
  Q : Outport
  wires:
  Delay/1 -> Inverter/1
  Inverter/1 -> Logical1/1
  Logical1/1 -> Q/1
  D/1 -> Delay/1, Logical1/2

== system wlan_agc/Ctrl/Posedge7 ==
  note: Rising Edge Detection
  D : Inport
  Delay : xbsIndex_r4/Delay  rst=off  infoeditControl=Selection of Reset will increase slice count due to use of real FFs and instead of SRLs  en=off  latency=1  dbl_ovrd=off  reg_retiming=off  block_type=delay
      settings: infoedit=Hardware notes: A delay line is a chain, each link of which is an SRL16 followed by a flip-flop. If register retiming is enabled, the delay line is a chain of flip-flops.  xl_area=[1 1 0 0 0 0 0]  block_version=VER_STRING_GOES_HERE
  Inverter : xbsIndex_r4/Inverter  en=off  latency=0  dbl_ovrd=off  block_type=inv
      settings: xl_area=[0 0 0 0 0 0 0]  block_version=VER_STRING_GOES_HERE
  Logical1 : xbsIndex_r4/Logical  logical_function=AND  inputs=2  en=off  latency=0  precision=Full  arith_type=Unsigned  n_bits=8  bin_pt=2  align_bp=on  dbl_ovrd=off  block_type=logical
      settings: xl_area=[1 0 0 1 0 0 0]  block_version=VER_STRING_GOES_HERE
  Q : Outport
  wires:
  Delay/1 -> Inverter/1
  Inverter/1 -> Logical1/1
  Logical1/1 -> Q/1
  D/1 -> Delay/1, Logical1/2

== system wlan_agc/Ctrl/Posedge8 ==
  note: Rising Edge Detection
  D : Inport
  Delay : xbsIndex_r4/Delay  rst=off  infoeditControl=Selection of Reset will increase slice count due to use of real FFs and instead of SRLs  en=off  latency=1  dbl_ovrd=off  reg_retiming=off  block_type=delay
      settings: infoedit=Hardware notes: A delay line is a chain, each link of which is an SRL16 followed by a flip-flop. If register retiming is enabled, the delay line is a chain of flip-flops.  xl_area=[1 1 0 0 0 0 0]  block_version=VER_STRING_GOES_HERE
  Inverter : xbsIndex_r4/Inverter  en=off  latency=0  dbl_ovrd=off  block_type=inv
      settings: xl_area=[0 0 0 0 0 0 0]  block_version=VER_STRING_GOES_HERE
  Logical1 : xbsIndex_r4/Logical  logical_function=AND  inputs=2  en=off  latency=0  precision=Full  arith_type=Unsigned  n_bits=8  bin_pt=2  align_bp=on  dbl_ovrd=off  block_type=logical
      settings: xl_area=[1 0 0 1 0 0 0]  block_version=VER_STRING_GOES_HERE
  Q : Outport
  wires:
  Delay/1 -> Inverter/1
  Inverter/1 -> Logical1/1
  Logical1/1 -> Q/1
  D/1 -> Delay/1, Logical1/2

== system wlan_agc/Ctrl/Posedge9 ==
  note: Rising Edge Detection
  D : Inport
  Delay : xbsIndex_r4/Delay  rst=off  infoeditControl=Selection of Reset will increase slice count due to use of real FFs and instead of SRLs  en=off  latency=1  dbl_ovrd=off  reg_retiming=off  block_type=delay
      settings: infoedit=Hardware notes: A delay line is a chain, each link of which is an SRL16 followed by a flip-flop. If register retiming is enabled, the delay line is a chain of flip-flops.  xl_area=[1 1 0 0 0 0 0]  block_version=VER_STRING_GOES_HERE
  Inverter : xbsIndex_r4/Inverter  en=off  latency=0  dbl_ovrd=off  block_type=inv
      settings: xl_area=[0 0 0 0 0 0 0]  block_version=VER_STRING_GOES_HERE
  Logical1 : xbsIndex_r4/Logical  logical_function=AND  inputs=2  en=off  latency=0  precision=Full  arith_type=Unsigned  n_bits=8  bin_pt=2  align_bp=on  dbl_ovrd=off  block_type=logical
      settings: xl_area=[1 0 0 1 0 0 0]  block_version=VER_STRING_GOES_HERE
  Q : Outport
  wires:
  D/1 -> Logical1/2, Delay/1
  Logical1/1 -> Q/1
  Inverter/1 -> Logical1/1
  Delay/1 -> Inverter/1

== system wlan_agc/Ctrl/Reset Counter ==
  IQ Valid : Inport
  Done : Inport  Port=2
  Constant2 : xbsIndex_r4/Constant  const=253  gui_display_data_type=Fixed-point  arith_type=Unsigned  n_bits=8  bin_pt=0  preci_type=Single  exp_width=8  frac_width=24  explicit_period=off  period=1  equ=P=C  opselect=C  inp2=PCIN>>17  opr=+  inp1=P  carry=CIN  dbl_ovrd=off  block_type=constant
      settings: block_version=VER_STRING_GOES_HERE
  Counter1 : xbsIndex_r4/Counter  cnt_type=Free Running  cnt_to=1023  operation=Up  start_count=0  cnt_by_val=1  arith_type=Unsigned  n_bits=8  bin_pt=0  load_pin=off  rst=on  en=on  explicit_period=off  period=1  dbl_ovrd=off  use_behavioral_HDL=off  implementation=Fabric  block_type=counter
  Inverter1 : xbsIndex_r4/Inverter  en=off  latency=0  dbl_ovrd=off  block_type=inv
      settings: xl_area=[0 0 0 0 0 0 0]  block_version=VER_STRING_GOES_HERE
  Logical2 : xbsIndex_r4/Logical  logical_function=AND  inputs=3  en=off  latency=0  precision=Full  arith_type=Unsigned  n_bits=16  bin_pt=0  align_bp=on  dbl_ovrd=off  block_type=logical
  Relational1 : xbsIndex_r4/Relational  mode=a<b  en=off  latency=0  dbl_ovrd=off  block_type=relational
  S-R Latch1 : Subsystem
  Count : Outport
  wires:
  Logical2/1 -> Counter1/2
  S-R Latch1/1(Q) -> Logical2/2
  Constant2/1 -> Relational1/2
  Relational1/1 -> Logical2/3, Inverter1/1
  Counter1/1 -> Relational1/1, Count/1
  Inverter1/1 -> Counter1/1, S-R Latch1/2(R)
  Done/1 -> S-R Latch1/1(S)
  IQ Valid/1 -> Logical2/1

== system wlan_agc/Ctrl/S-R Latch ==
  S : Inport
  R : Inport  Port=2
  Constant1 : xbsIndex_r4/Constant  const=1  gui_display_data_type=Boolean  arith_type=Boolean  n_bits=1  bin_pt=0  preci_type=Single  exp_width=8  frac_width=24  explicit_period=off  period=1  equ=P=C  opselect=C  inp2=PCIN>>17  opr=+  inp1=P  carry=CIN  dbl_ovrd=off  block_type=constant
      settings: block_version=VER_STRING_GOES_HERE
  Convert1 : xbsIndex_r4/Convert  gui_display_data_type=Boolean  arith_type=Boolean  n_bits=1  bin_pt=0  float_type=Single  exp_bits=8  fraction_bits=24  quantization=Truncate  overflow=Wrap  en=off  latency=0  dbl_ovrd=off  pipeline=off  block_type=convert
  Convert2 : xbsIndex_r4/Convert  gui_display_data_type=Boolean  arith_type=Boolean  n_bits=1  bin_pt=0  float_type=Single  exp_bits=8  fraction_bits=24  quantization=Truncate  overflow=Wrap  en=off  latency=0  dbl_ovrd=off  pipeline=off  block_type=convert
  Register2 : xbsIndex_r4/Register  init=0  rst=on  en=on  dbl_ovrd=off  block_type=register
      settings: xl_area=[1 1 0 0 0 0 0]  block_version=VER_STRING_GOES_HERE
  Q : Outport
  wires:
  Convert2/1 -> Register2/3
  Convert1/1 -> Register2/2
  Constant1/1 -> Register2/1
  R/1 -> Convert1/1
  Register2/1 -> Q/1
  S/1 -> Convert2/1

== system wlan_agc/Ctrl/Start Counter ==
  IQ Valid : Inport
  Start : Inport  Port=2
  Done : Inport  Port=3
  Constant1 : xbsIndex_r4/Constant  const=253  gui_display_data_type=Fixed-point  arith_type=Unsigned  n_bits=8  bin_pt=0  preci_type=Single  exp_width=8  frac_width=24  explicit_period=off  period=1  equ=P=C  opselect=C  inp2=PCIN>>17  opr=+  inp1=P  carry=CIN  dbl_ovrd=off  block_type=constant
      settings: block_version=VER_STRING_GOES_HERE
  Counter : xbsIndex_r4/Counter  cnt_type=Free Running  cnt_to=1023  operation=Up  start_count=0  cnt_by_val=1  arith_type=Unsigned  n_bits=8  bin_pt=0  load_pin=off  rst=on  en=on  explicit_period=off  period=1  dbl_ovrd=off  use_behavioral_HDL=off  implementation=Fabric  block_type=counter
  Inverter : xbsIndex_r4/Inverter  en=off  latency=0  dbl_ovrd=off  block_type=inv
      settings: xl_area=[0 0 0 0 0 0 0]  block_version=VER_STRING_GOES_HERE
  Logical : xbsIndex_r4/Logical  logical_function=AND  inputs=3  en=off  latency=0  precision=Full  arith_type=Unsigned  n_bits=16  bin_pt=0  align_bp=on  dbl_ovrd=off  block_type=logical
  Logical1 : xbsIndex_r4/Logical  logical_function=OR  inputs=2  en=off  latency=0  precision=Full  arith_type=Unsigned  n_bits=16  bin_pt=0  align_bp=on  dbl_ovrd=off  block_type=logical
  Relational5 : xbsIndex_r4/Relational  mode=a<b  en=off  latency=0  dbl_ovrd=off  block_type=relational
  S-R Latch : Subsystem
  Count : Outport
  tag scope: AGC_RESET=global
  wires:
  S-R Latch/1(Q) -> Logical/1, Inverter/1
  Logical/1 -> Counter/2
  Inverter/1 -> Counter/1, [AGC_RESET]
  Logical1/1 -> S-R Latch/2(R)
  [reg_AGC_RESET] -> Logical1/2
  Counter/1 -> Relational5/1, Count/1
  Relational5/1 -> Logical/3
  Constant1/1 -> Relational5/2
  Done/1 -> Logical1/1
  Start/1 -> S-R Latch/1(S)
  IQ Valid/1 -> Logical/2

== system wlan_agc/DCO Correction/DCO Corr ==
  IQ Valid : Inport
  I : Inport  Port=2
  Q : Inport  Port=3
  Accumulator : xbsIndex_r4/Accumulator  operation=Add  n_bits=17  overflow=Flag as error  scale=1  rst=on  infoeditControl=reset for floating point data type must be asserted for a minimum of 2 cycles  hasbypass=off  en=on  latency=0  dbl_ovrd=off  msb_inp=100  msb=100  lsb=-100  use_behavioral_HDL=on  implementation=Fabric  block_type=accum
      settings: block_version=VER_STRING_GOES_HERE
  Accumulator1 : xbsIndex_r4/Accumulator  operation=Add  n_bits=17  overflow=Flag as error  scale=1  rst=on  infoeditControl=reset for floating point data type must be asserted for a minimum of 2 cycles  hasbypass=off  en=on  latency=0  dbl_ovrd=off  msb_inp=100  msb=100  lsb=-100  use_behavioral_HDL=on  implementation=Fabric  block_type=accum
      settings: block_version=VER_STRING_GOES_HERE
  AddSub : xbsIndex_r4/AddSub  mode=Subtraction  use_carryin=off  use_carryout=off  en=off  latency=1  precision=User Defined  arith_type="Signed  (2's comp)"  n_bits=16  bin_pt=15  quantization=Truncate  overflow=Wrap  dbl_ovrd=off  use_behavioral_HDL=off  hw_selection=Fabric  pipelined=off  block_type=addsub
  AddSub1 : xbsIndex_r4/AddSub  mode=Subtraction  use_carryin=off  use_carryout=off  en=off  latency=1  precision=User Defined  arith_type="Signed  (2's comp)"  n_bits=16  bin_pt=15  quantization=Truncate  overflow=Wrap  dbl_ovrd=off  use_behavioral_HDL=off  hw_selection=Fabric  pipelined=off  block_type=addsub
  Constant : xbsIndex_r4/Constant  const=31  gui_display_data_type=Fixed-point  arith_type=Unsigned  n_bits=5  bin_pt=0  preci_type=Single  exp_width=8  frac_width=24  explicit_period=off  period=1  equ=P=C  opselect=C  inp2=PCIN>>17  opr=+  inp1=P  carry=CIN  dbl_ovrd=off  block_type=constant
  Counter : xbsIndex_r4/Counter  cnt_type=Free Running  cnt_to=Inf  operation=Up  start_count=0  cnt_by_val=1  arith_type=Unsigned  n_bits=5  bin_pt=0  load_pin=off  rst=on  en=on  explicit_period=off  period=1  dbl_ovrd=off  use_behavioral_HDL=off  implementation=Fabric  block_type=counter
  DCO Est : Scope  NumInputPorts=7
      settings: TimeRange=10000  YMin=-0.4~-0.4~0~0~-0.02~-0.4~-0.4  YMax=0.4~0.4~1~0.03~0.009999999999999999~0.4~0.4
  Delay : xbsIndex_r4/Delay  rst=off  infoeditControl=Selection of Reset will increase slice count due to use of real FFs and instead of SRLs  en=off  latency=1  dbl_ovrd=off  reg_retiming=off  block_type=delay
  Logical : xbsIndex_r4/Logical  logical_function=AND  inputs=2  en=off  latency=0  precision=Full  arith_type=Unsigned  n_bits=16  bin_pt=0  align_bp=on  dbl_ovrd=off  block_type=logical
  Logical1 : xbsIndex_r4/Logical  logical_function=OR  inputs=2  en=off  latency=0  precision=Full  arith_type=Unsigned  n_bits=16  bin_pt=0  align_bp=on  dbl_ovrd=off  block_type=logical
  Logical2 : xbsIndex_r4/Logical  logical_function=AND  inputs=2  en=off  latency=0  precision=Full  arith_type=Unsigned  n_bits=16  bin_pt=0  align_bp=on  dbl_ovrd=off  block_type=logical
  Relational : xbsIndex_r4/Relational  mode=a=b  en=off  latency=0  dbl_ovrd=off  block_type=relational
  S-R Latch : Subsystem
  Scale : xbsIndex_r4/Scale  scale_factor=-5  dbl_ovrd=off  block_type=scale
  Scale1 : xbsIndex_r4/Scale  scale_factor=-5  dbl_ovrd=off  block_type=scale
  done{1..7} (7 alike) : xbsIndex_r4/Gateway Out  inherit_from_input=off  hdl_port=off  timing_constraint=None  locs_specified=off  LOCs={}  UseAsDAC=off  DACChannel='1'  block_type=gatewayout
      settings: infoedit="Gateway out block.  Converts Xilinx fixed point inputs into ouputs of type Simulink integer, double, or fixed point.<P><P>Hardware notes:  In hardware these blocks become top level output ports or are discarded, depending on how they are configured."  xl_area=[0 0 0 0 1 0 0]  block_version=VER_STRING_GOES_HERE
  Valid : Outport
  " I" : Outport  Port=2
  " Q" : Outport  Port=3
  wires:
  I/1 -> Accumulator/1, AddSub/1, done4/1
  Q/1 -> Accumulator1/1, AddSub1/1, done2/1
  [AGC_RESET] -> Accumulator1/2, Accumulator/2
  [AGC_CTRL_Start_DCO] -> S-R Latch/1(S)
  Logical/1 -> Counter/2, Accumulator1/3, Accumulator/3, done5/1
  Constant/1 -> Relational/2
  Counter/1 -> Relational/1
  S-R Latch/1(Q) -> Logical/2
  IQ Valid/1 -> Delay/1, Logical/1, Logical2/1
  Accumulator/1 -> Scale/1
  Accumulator1/1 -> Scale1/1
  [AGC_RESET] -> Logical1/1
  Logical1/1 -> S-R Latch/2(R), Counter/1
  AddSub/1 -> " I"/1, done1/1
  AddSub1/1 -> " Q"/1, done7/1
  Delay/1 -> Valid/1
  Relational/1 -> Logical2/2
  Logical2/1 -> Logical1/2
  Scale/1 -> AddSub/2, done3/1
  Scale1/1 -> AddSub1/2, done6/1
  done4/1 -> DCO Est/1
  done2/1 -> DCO Est/2
  done6/1 -> DCO Est/5
  done5/1 -> DCO Est/3
  done3/1 -> DCO Est/4
  done1/1 -> DCO Est/6
  done7/1 -> DCO Est/7
